simulink library "prj5pelib"  (R2021a)
settings: Solver=VariableStepAuto  StartTime=0.0  StopTime=10.0  RelTol=1e-3
libraries: hdlBasic x7
settings Model: Creator=asc8  LastModifiedBy=asc8

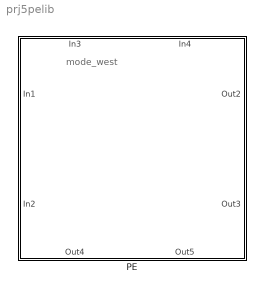
== system prj5pelib ==
  note: mode_west
  PE : Subsystem
      settings: PortSchema="{\"entries\":[{\"content\":{\"sides\":[{\"content\":{\"connectorIds\":[\"In1\",\"In2\"]},\"type\":\"ConnectorPlacement.EquallySpacedRectSide\",\"uuid\":\"f7e55443-70fb-4ed5-ab4f-147f7311106a\"},{\"content\":{\"connectorIds\":[\"Out1\",\"Out2\"],\"side\":\"RIGHT\"},\"type\":\"ConnectorPlacement.EquallySpacedRectSide\",\"uuid\":\"6de0769a-4a22-4abb-b630-26d0c175204f\"},{\"content\":{\"connectorIds\":[\"In3\",\"In4\"],\"side\":\"TOP\"},\"type\":\"ConnectorPlacement.EquallySpacedRectSide\",\"uuid\":\"a041cc58-78e8-4444-b053-dd6f2c27badd\"},{\"content\":{\"connectorIds\":[\"Out3\",\"Out4\"],\"side\":\"BOTTOM\"},\"type\":\"ConnectorPlacement.EquallySpacedRectSide\",\"uuid\":\"085ff6f5-8624-4aab-b622-9beedcd77ebd\"}]},\"type\":\"ConnectorPlacement.EquallySpacedConnector\",\"uuid\":\"928950cd-8b9e-4ebf-b8fd-b98c3e494fdc\"}],\"packageUris\":[\"http://schema.mathworks.com/mf0/Connector/R2020b\"],\"version\":\"1.0\"}"

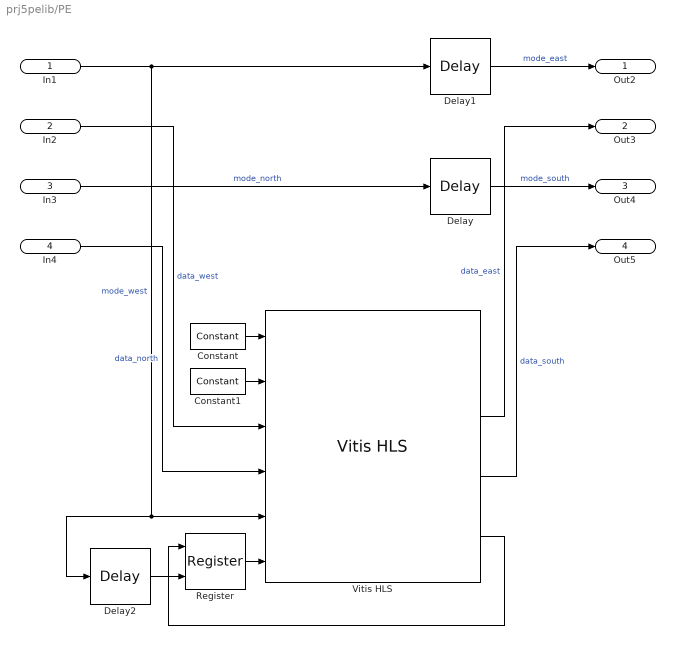
== system prj5pelib/PE ==
  In1 : Inport
  In2 : Inport  Port=2
  In3 : Inport  Port=3
  In4 : Inport  Port=4
  Constant : hdlBasic/Constant  const=0  gui_display_data_type=Boolean  arith_type=Boolean  n_bits=16  bin_pt=14  preci_type=Single  exp_width=8  frac_width=24  explicit_period=on  period=1  XmcBlockStatus=1  maskContainerNames=tabcontainer1  block_type=constant  block_config=sysgen:Constant_config
  Constant1 : hdlBasic/Constant  const=1  gui_display_data_type=Boolean  arith_type=Boolean  n_bits=16  bin_pt=14  preci_type=Single  exp_width=8  frac_width=24  explicit_period=on  period=1  XmcBlockStatus=1  maskContainerNames=tabcontainer1  block_type=constant  block_config=sysgen:Constant_config
  Delay : hdlBasic/Delay  rst=off  en=off  latency=20  reg_retiming=off  XmcBlockStatus=1  maskContainerNames=group1  block_type=delay  block_config=sysgen:Delay_config
  Delay1 : hdlBasic/Delay  rst=off  en=off  latency=20  reg_retiming=off  XmcBlockStatus=1  maskContainerNames=group1  block_type=delay  block_config=sysgen:Delay_config
  Delay2 : hdlBasic/Delay  rst=off  en=off  latency=1  reg_retiming=off  XmcBlockStatus=1  maskContainerNames=group1  block_type=delay  block_config=sysgen:Delay_config
  Register : hdlBasic/Register  init=0  rst=off  en=on  XmcBlockStatus=1  maskContainerNames=tabcontainer1  block_type=register  block_config=sysgen:Register_config
  Vitis HLS : hdlBasic/Vitis HLS  anytable='.\Vitis_HLS\cordic_raw\solution1'  fast_sim=off  display_datatype=off  rate_propagation_method=Simulink system period  model_file_path=''  latency=1  block_type=vitis_hls
      settings: infoedit=This block allows including C,C++ and SystemC source files in System Generator for DSP designs.
  Out2 : Outport
  Out3 : Outport  Port=2
  Out4 : Outport  Port=3
  Out5 : Outport  Port=4
  wires:
  In3/1 -> Delay/1  "mode_north"
  In4/1 -> Vitis HLS/4  "data_north"
  In1/1 -> Delay1/1, Delay2/1, Vitis HLS/5  "mode_west"
  In2/1 -> Vitis HLS/3  "data_west"
  Delay1/1 -> Out2/1  "mode_east"
  Vitis HLS/4 -> Out3/1  "data_east"
  Delay/1 -> Out4/1  "mode_south"
  Vitis HLS/6 -> Out5/1  "data_south"
  Constant/1 -> Vitis HLS/1
  Constant1/1 -> Vitis HLS/2
  Register/1 -> Vitis HLS/6
  Vitis HLS/8 -> Register/1
  Delay2/1 -> Register/2
